simulink model "Control_try_final_2020b"  (R2020b)
settings: Solver=VariableStepAuto  StartTime=0.0  StopTime=inf  RelTol=1e-3
undefined symbols (not defined in the file or in its folder): DiscIntNeverNeededParam
libraries: mobileRoboticsLib x25
(part 2 of 7)

== system Control_try_final_2020b/Team_1_behaviour/T1R2 (attacker 1) ==
  R_1_loc : Inport
  R_2_loc : Inport  Port=2
  R_4_loc : Inport  Port=3
  R_3_loc : Inport  Port=4
  Ball Loc : Inport  Port=5
  R_2_sen : Inport  Port=6
  reset : Inport  Port=7
  did_goal : Inport  Port=8
  foul_team_right : Inport  Port=9
  foul_team_left : Inport  Port=10
  throwin_foul_loc : Inport  Port=11
  Chart1 : Stateflow chart  TreatAsAtomicUnit=on
      settings: PortSchema="{\"entries\":[{\"content\":{\"sides\":[{\"content\":{\"connectorIds\":[\"In8\",\"In2\",\"In3\",\"In4\",\"In5\",\"In6\",\"In7\",\"In9\"]},\"type\":\"ConnectorPlacement.EquallySpacedRectSide\",\"uuid\":\"fbe3839a-d39c-4c99-9a0b-e35240c09fc7\"},{\"content\":{\"connectorIds\":[\"Out1\",\"Out2\",\"Out3\"],\"side\":\"RIGHT\"},\"type\":\"ConnectorPlacement.EquallySpacedRectSide\",\"uuid\":\"d50292e7-ec87-4cb2-bfda-821c8e119e63\"},{\"content\":{\"connectorIds\":[\"In1\"],\"side\":\"TOP\"},\"type\":\"ConnectorPlacement.EquallySpacedRectSide\",\"uuid\":\"096c229a-97d6-46f3-b3a2-f22035fee078\"}]},\"type\":\"ConnectorPlacement.EquallySpacedConnector\",\"uuid\":\"90e2ed61-57b9-4a5d-b9f9-31cf1ac9de3f\"}],\"packageUris\":[\"http://schema.mathworks.com/mf0/Connector/R2020b\"],\"version\":\"1.0\"}"
  Demux : Demux  Outputs=3
  Demux1 : Demux  Outputs=2
  IC1 : InitialCondition  Value=[0;0;0]
  Team 1 Behaviour1 : Subsystem
      settings: PortSchema="{\"entries\":[{\"content\":{\"sides\":[{\"content\":{\"connectorIds\":[]},\"type\":\"ConnectorPlacement.EquallySpacedRectSide\",\"uuid\":\"be901545-21b9-45e5-bac5-a8cb9027aef5\"},{\"content\":{\"connectorIds\":[\"In1\",\"In2\",\"In3\",\"Out1\",\"Out2\",\"In4\",\"In5\",\"In6\",\"In7\",\"In8\"],\"side\":\"RIGHT\"},\"type\":\"ConnectorPlacement.EquallySpacedRectSide\",\"uuid\":\"b7c1eb84-2f14-4c7f-a74c-d56efbe0743e\"},{\"content\":{\"connectorIds\":[],\"side\":\"TOP\"},\"type\":\"ConnectorPlacement.EquallySpacedRectSide\",\"uuid\":\"aca41723-ed3f-4bd2-8fc1-457d075e3460\"}]},\"type\":\"ConnectorPlacement.EquallySpacedConnector\",\"uuid\":\"e10e22f1-c8f0-4dfc-85d2-4ba01528372d\"}],\"packageUris\":[\"http://schema.mathworks.com/mf0/Connector/R2020b\"],\"version\":\"1.0\"}"
  VxVyW : Outport
  XYZK : Outport  Port=2
  wires:
  R_2_sen/1 -> Team 1 Behaviour1/5(Robot 7 sens)
  R_4_loc/1 -> Team 1 Behaviour1/7(Robot 6 T1 Loc3)
  R_1_loc/1 -> Team 1 Behaviour1/8(Robot 5 T1 Loc4)
  R_3_loc/1 -> Team 1 Behaviour1/6(Robot 8 T1 Loc2)
  Demux1/2 -> Chart1/7(foul_loc_y)
  R_2_loc/1 -> Team 1 Behaviour1/4(Robot 1 T1 Loc), Chart1/1(R_2_loc)
  Demux1/1 -> Chart1/6(foul_loc_x)
  Demux/1 -> Chart1/2(bx)
  throwin_foul_loc/1 -> Demux1/1
  Ball Loc/1 -> Demux/1
  foul_team_left/1 -> Chart1/5(foul_team_left)
  did_goal/1 -> Chart1/9(did_goal)
  foul_team_right/1 -> Chart1/4(foul_team_right)
  Demux/2 -> Chart1/3(by)
  Chart1/3(velocity_UA) -> Team 1 Behaviour1/1(velocity_UA)
  Team 1 Behaviour1/1(XYZK) -> XYZK/1
  reset/1 -> Chart1/8(reset)
  Chart1/1(dest) -> IC1/1
  IC1/1 -> Team 1 Behaviour1/3(Ball Loc)
  Team 1 Behaviour1/2(VxVyW) -> VxVyW/1
  Chart1/2(kick_UA) -> Team 1 Behaviour1/2(kick_UA)

== system Control_try_final_2020b/Team_1_behaviour/T1R3 (Defender 2) ==
  R_1_loc : Inport
  R_2_loc : Inport  Port=2
  R_4_loc : Inport  Port=3
  R_3_loc : Inport  Port=4
  Ball Loc : Inport  Port=5
  reset : Inport  Port=6
  R_4_sen : Inport  Port=7
  did_goal : Inport  Port=8
  foul_team_right : Inport  Port=9
  foul_team_left : Inport  Port=10
  throwin_foul_loc : Inport  Port=11
  Chart : Stateflow chart  TreatAsAtomicUnit=on
      settings: PortSchema="{\"entries\":[{\"content\":{\"sides\":[{\"content\":{\"connectorIds\":[\"In9\",\"In2\",\"In3\",\"In4\",\"In5\",\"In6\",\"In7\",\"In8\"]},\"type\":\"ConnectorPlacement.EquallySpacedRectSide\",\"uuid\":\"fbe3839a-d39c-4c99-9a0b-e35240c09fc7\"},{\"content\":{\"connectorIds\":[\"Out1\",\"Out2\",\"Out3\"],\"side\":\"RIGHT\"},\"type\":\"ConnectorPlacement.EquallySpacedRectSide\",\"uuid\":\"d50292e7-ec87-4cb2-bfda-821c8e119e63\"},{\"content\":{\"connectorIds\":[\"In1\"],\"side\":\"TOP\"},\"type\":\"ConnectorPlacement.EquallySpacedRectSide\",\"uuid\":\"096c229a-97d6-46f3-b3a2-f22035fee078\"}]},\"type\":\"ConnectorPlacement.EquallySpacedConnector\",\"uuid\":\"90e2ed61-57b9-4a5d-b9f9-31cf1ac9de3f\"}],\"packageUris\":[\"http://schema.mathworks.com/mf0/Connector/R2020b\"],\"version\":\"1.0\"}"
  Demux : Demux  Outputs=3
  Demux1 : Demux  Outputs=2
  IC : InitialCondition  Value=[0;0;0]
  Team 1 Behaviour1 : Subsystem
      settings: PortSchema="{\"entries\":[{\"content\":{\"sides\":[{\"content\":{\"connectorIds\":[]},\"type\":\"ConnectorPlacement.EquallySpacedRectSide\",\"uuid\":\"be901545-21b9-45e5-bac5-a8cb9027aef5\"},{\"content\":{\"connectorIds\":[\"In1\",\"In2\",\"In3\",\"Out1\",\"Out2\",\"In4\",\"In5\",\"In6\",\"In7\",\"In8\"],\"side\":\"RIGHT\"},\"type\":\"ConnectorPlacement.EquallySpacedRectSide\",\"uuid\":\"b7c1eb84-2f14-4c7f-a74c-d56efbe0743e\"},{\"content\":{\"connectorIds\":[],\"side\":\"TOP\"},\"type\":\"ConnectorPlacement.EquallySpacedRectSide\",\"uuid\":\"aca41723-ed3f-4bd2-8fc1-457d075e3460\"}]},\"type\":\"ConnectorPlacement.EquallySpacedConnector\",\"uuid\":\"e10e22f1-c8f0-4dfc-85d2-4ba01528372d\"}],\"packageUris\":[\"http://schema.mathworks.com/mf0/Connector/R2020b\"],\"version\":\"1.0\"}"
  XYZK : Outport
  Out2 : Outport  Port=2
  wires:
  R_4_sen/1 -> Team 1 Behaviour1/5(Robot 7 sens)
  R_2_loc/1 -> Team 1 Behaviour1/7(Robot 6 T1 Loc3)
  R_3_loc/1 -> Team 1 Behaviour1/6(Robot 8 T1 Loc2)
  R_1_loc/1 -> Team 1 Behaviour1/8(Robot 5 T1 Loc4)
  foul_team_right/1 -> Chart/4(foul_team_right)
  throwin_foul_loc/1 -> Demux1/1
  Demux1/2 -> Chart/8(foul_loc_y)
  Demux1/1 -> Chart/7(foul_loc_x)
  did_goal/1 -> Chart/6(did_goal)
  foul_team_left/1 -> Chart/5(foul_team_left)
  Demux/2 -> Chart/3(by)
  Chart/3(velocity_UA) -> Team 1 Behaviour1/1(velocity_UA)
  Chart/1(dest) -> IC/1
  Chart/2(kick_UA) -> Team 1 Behaviour1/2(kick_UA)
  Team 1 Behaviour1/2(VxVyW) -> XYZK/1
  Demux/1 -> Chart/2(bx)
  IC/1 -> Team 1 Behaviour1/3(Ball Loc)
  Team 1 Behaviour1/1(XYZK) -> Out2/1
  reset/1 -> Chart/9(reset)
  R_4_loc/1 -> Team 1 Behaviour1/4(Robot 1 T1 Loc), Chart/1(R_2_loc)
  Ball Loc/1 -> Demux/1

== system Control_try_final_2020b/Team_1_behaviour/T1R3 (defender 1) ==
  R_1_loc : Inport
  R_2_loc : Inport  Port=2
  R_4_loc : Inport  Port=3
  R_3_loc : Inport  Port=4
  Ball Loc : Inport  Port=5
  reset : Inport  Port=6
  R_3_sen : Inport  Port=7
  did_goal : Inport  Port=8
  foul_team_right : Inport  Port=9
  foul_team_left : Inport  Port=10
  throwin_foul_loc : Inport  Port=11
  Chart : Stateflow chart  TreatAsAtomicUnit=on
      settings: PortSchema="{\"entries\":[{\"content\":{\"sides\":[{\"content\":{\"connectorIds\":[\"In8\",\"In2\",\"In3\",\"In4\",\"In5\",\"In6\",\"In7\",\"In9\"]},\"type\":\"ConnectorPlacement.EquallySpacedRectSide\",\"uuid\":\"fbe3839a-d39c-4c99-9a0b-e35240c09fc7\"},{\"content\":{\"connectorIds\":[\"Out1\",\"Out2\",\"Out3\"],\"side\":\"RIGHT\"},\"type\":\"ConnectorPlacement.EquallySpacedRectSide\",\"uuid\":\"d50292e7-ec87-4cb2-bfda-821c8e119e63\"},{\"content\":{\"connectorIds\":[\"In1\"],\"side\":\"TOP\"},\"type\":\"ConnectorPlacement.EquallySpacedRectSide\",\"uuid\":\"096c229a-97d6-46f3-b3a2-f22035fee078\"},{\"content\":{\"connectorIds\":[],\"side\":\"BOTTOM\"},\"type\":\"ConnectorPlacement.EquallySpacedRectSide\",\"uuid\":\"82b7a600-d24c-4262-afa5-d1d8e08c64b1\"}]},\"type\":\"ConnectorPlacement.EquallySpacedConnector\",\"uuid\":\"90e2ed61-57b9-4a5d-b9f9-31cf1ac9de3f\"}],\"packageUris\":[\"http://schema.mathworks.com/mf0/Connector/R2020b\"],\"version\":\"1.0\"}"
  Demux : Demux  Outputs=3
  Demux1 : Demux  Outputs=2
  IC : InitialCondition  Value=[0;0;0]
  Team 1 Behaviour : Subsystem  Commented=on
      settings: PortSchema="{\"entries\":[{\"content\":{\"sides\":[{\"content\":{\"connectorIds\":[]},\"type\":\"ConnectorPlacement.EquallySpacedRectSide\",\"uuid\":\"be901545-21b9-45e5-bac5-a8cb9027aef5\"},{\"content\":{\"connectorIds\":[\"In1\",\"Out1\",\"Out2\",\"In2\"],\"side\":\"RIGHT\"},\"type\":\"ConnectorPlacement.EquallySpacedRectSide\",\"uuid\":\"b7c1eb84-2f14-4c7f-a74c-d56efbe0743e\"},{\"content\":{\"connectorIds\":[],\"side\":\"TOP\"},\"type\":\"ConnectorPlacement.EquallySpacedRectSide\",\"uuid\":\"aca41723-ed3f-4bd2-8fc1-457d075e3460\"}]},\"type\":\"ConnectorPlacement.EquallySpacedConnector\",\"uuid\":\"e10e22f1-c8f0-4dfc-85d2-4ba01528372d\"}],\"packageUris\":[\"http://schema.mathworks.com/mf0/Connector/R2020b\"],\"version\":\"1.0\"}"
  Team 1 Behaviour1 : Subsystem
      settings: PortSchema="{\"entries\":[{\"content\":{\"sides\":[{\"content\":{\"connectorIds\":[]},\"type\":\"ConnectorPlacement.EquallySpacedRectSide\",\"uuid\":\"be901545-21b9-45e5-bac5-a8cb9027aef5\"},{\"content\":{\"connectorIds\":[\"In1\",\"In2\",\"In3\",\"Out1\",\"Out2\",\"In4\",\"In5\",\"In6\",\"In7\",\"In8\"],\"side\":\"RIGHT\"},\"type\":\"ConnectorPlacement.EquallySpacedRectSide\",\"uuid\":\"b7c1eb84-2f14-4c7f-a74c-d56efbe0743e\"},{\"content\":{\"connectorIds\":[],\"side\":\"TOP\"},\"type\":\"ConnectorPlacement.EquallySpacedRectSide\",\"uuid\":\"aca41723-ed3f-4bd2-8fc1-457d075e3460\"}]},\"type\":\"ConnectorPlacement.EquallySpacedConnector\",\"uuid\":\"e10e22f1-c8f0-4dfc-85d2-4ba01528372d\"}],\"packageUris\":[\"http://schema.mathworks.com/mf0/Connector/R2020b\"],\"version\":\"1.0\"}"
  VxVyW : Outport
  XYZK : Outport  Port=2
  wires:
  reset/1 -> Chart/8(reset)
  Ball Loc/1 -> Demux/1
  Demux/1 -> Chart/2(bx)
  Team 1 Behaviour1/2(VxVyW) -> VxVyW/1
  Team 1 Behaviour1/1(XYZK) -> XYZK/1
  R_3_loc/1 -> Team 1 Behaviour1/4(Robot 1 T1 Loc), Chart/1(R_2_loc)
  Demux/2 -> Chart/3(by)
  Chart/1(dest) -> IC/1
  IC/1 -> Team 1 Behaviour1/3(Ball Loc)
  Chart/2(kick_UA) -> Team 1 Behaviour1/2(kick_UA)
  Chart/3(velocity_UA) -> Team 1 Behaviour1/1(velocity_UA)
  did_goal/1 -> Chart/9(did_goal)
  foul_team_right/1 -> Chart/7(foul_team_right)
  foul_team_left/1 -> Chart/4(foul_team_left)
  throwin_foul_loc/1 -> Demux1/1
  Demux1/1 -> Chart/5(foul_loc_x)
  Demux1/2 -> Chart/6(foul_loc_y)
  R_1_loc/1 -> Team 1 Behaviour1/8(Robot 5 T1 Loc4)
  R_3_sen/1 -> Team 1 Behaviour1/5(Robot 7 sens)
  R_2_loc/1 -> Team 1 Behaviour1/7(Robot 6 T1 Loc3)
  R_4_loc/1 -> Team 1 Behaviour1/6(Robot 8 T1 Loc2)

== system Control_try_final_2020b/Team_2_Behaviour/T2_R1(Goal_Keeper) ==
  R_1_loc : Inport
  R_2_loc : Inport  Port=2
  R_4_loc : Inport  Port=3
  R_3_loc : Inport  Port=4
  Ball Loc : Inport  Port=5
  R_1_sen : Inport  Port=6
  Constant : Constant  Value=0
  Constant1 : Constant  Value=0
  Demux : Demux  Outputs=3
  Demux1 : Demux  Outputs=3
  Display : Display
  Distance : Subsystem
      settings: PortSchema="{\"entries\":[{\"content\":{\"sides\":[{\"content\":{\"connectorIds\":[]},\"type\":\"ConnectorPlacement.EquallySpacedRectSide\",\"uuid\":\"931fdb8b-3711-4e7f-9cbc-53e0dea53fca\"},{\"content\":{\"connectorIds\":[\"Out1\"],\"side\":\"RIGHT\"},\"type\":\"ConnectorPlacement.EquallySpacedRectSide\",\"uuid\":\"ee0c7800-c700-48d1-aa4f-dd4a30624bbc\"},{\"content\":{\"connectorIds\":[\"In1\",\"In2\"],\"side\":\"TOP\"},\"type\":\"ConnectorPlacement.EquallySpacedRectSide\",\"uuid\":\"9579cc4b-8b33-4755-9564-e19cfe104d2b\"},{\"content\":{\"connectorIds\":[\"In3\",\"In4\"],\"side\":\"BOTTOM\"},\"type\":\"ConnectorPlacement.EquallySpacedRectSide\",\"uuid\":\"3469c1a3-363b-4534-8624-9a42e1898f6f\"}]},\"type\":\"ConnectorPlacement.EquallySpacedConnector\",\"uuid\":\"efd995f2-e999-4310-9f3f-88c38333e880\"}],\"packageUris\":[\"http://schema.mathworks.com/mf0/Connector/R2020b\"],\"version\":\"1.0\"}"
  Vector Concatenate : Concatenate  NumInputs=3
  angle_finder : Subsystem
  control : Stateflow chart  TreatAsAtomicUnit=on
      settings: PortSchema="{\"entries\":[{\"content\":{\"sides\":[{\"content\":{\"connectorIds\":[\"In1\",\"In4\",\"In3\",\"In2\",\"In5\"]},\"type\":\"ConnectorPlacement.EquallySpacedRectSide\",\"uuid\":\"fa0fd246-e6b9-4dd4-94af-e6e1e45d6f7d\"},{\"content\":{\"connectorIds\":[\"Out1\",\"Out2\"],\"side\":\"RIGHT\"},\"type\":\"ConnectorPlacement.EquallySpacedRectSide\",\"uuid\":\"3f196244-96d1-41e4-aa84-a415e0f99109\"},{\"content\":{\"connectorIds\":[],\"side\":\"TOP\"},\"type\":\"ConnectorPlacement.EquallySpacedRectSide\",\"uuid\":\"731ebc3a-62ab-4275-8d10-19257bb8fb52\"}]},\"type\":\"ConnectorPlacement.EquallySpacedConnector\",\"uuid\":\"dccf28de-3df1-4952-8544-1d4b47a347e5\"}],\"packageUris\":[\"http://schema.mathworks.com/mf0/Connector/R2020b\"],\"version\":\"1.0\"}"
  min_Distance_Finder : Subsystem
      settings: PortSchema="{\"entries\":[{\"content\":{\"sides\":[{\"content\":{\"connectorIds\":[\"In1\",\"In2\"]},\"type\":\"ConnectorPlacement.EquallySpacedRectSide\",\"uuid\":\"45cf91c7-7d38-4a19-bf35-d1d31095287a\"},{\"content\":{\"connectorIds\":[\"Out1\"],\"side\":\"RIGHT\"},\"type\":\"ConnectorPlacement.EquallySpacedRectSide\",\"uuid\":\"645394ba-2e5d-4060-b61c-cc9330ee0038\"},{\"content\":{\"connectorIds\":[\"In3\",\"In4\",\"In5\"],\"side\":\"TOP\"},\"type\":\"ConnectorPlacement.EquallySpacedRectSide\",\"uuid\":\"4fc56b73-04ec-476f-b487-f0e593f708ad\"},{\"content\":{\"connectorIds\":[],\"side\":\"BOTTOM\"},\"type\":\"ConnectorPlacement.EquallySpacedRectSide\",\"uuid\":\"cd306436-fd63-4e79-88e6-7a63c0840ed7\"}]},\"type\":\"ConnectorPlacement.EquallySpacedConnector\",\"uuid\":\"5cf2ee04-00eb-490b-958c-5fb90b43d325\"}],\"packageUris\":[\"http://schema.mathworks.com/mf0/Connector/R2020b\"],\"version\":\"1.0\"}"
  R1_vel_Y : Outport
  kick : Outport  Port=2  PortDimensions=4
  wires:
  Ball Loc/1 -> Demux/1
  Demux/2 -> control/5(Ball_loc_Y), Distance/4(In4)
  R_1_loc/1 -> Demux1/1, angle_finder/2(R_1_loc), min_Distance_Finder/2(R_1_loc)
  Demux1/2 -> control/4(R1_loc_Y), Distance/2(In2)
  Demux1/1 -> control/1(R1_loc_X), Distance/1(In1)
  R_2_loc/1 -> min_Distance_Finder/3(R_2_loc)
  R_3_loc/1 -> min_Distance_Finder/4(R_3_loc)
  R_4_loc/1 -> min_Distance_Finder/5(R_4_loc)
  R_1_sen/1 -> min_Distance_Finder/1(R_1_sen)
  Demux/1 -> control/2(Ball_loc_X), Distance/3(In3)
  control/2(R1_vel_Y) -> Vector Concatenate/2
  Distance/1(GB_dist) -> control/3(GB_dist)
  Vector Concatenate/1 -> R1_vel_Y/1
  Constant/1 -> Vector Concatenate/1
  Constant1/1 -> Vector Concatenate/3
  min_Distance_Finder/1(kick_direction) -> angle_finder/1(kick_direction)
  control/1(kick) -> angle_finder/3(kick)
  angle_finder/1(Out1) -> Display/1, kick/1

== system Control_try_final_2020b/Team_2_Behaviour/T2_R2(defender) ==
  R_1_loc : Inport
  R_2_loc : Inport  Port=2
  R_4_loc : Inport  Port=3
  R_3_loc : Inport  Port=4
  Ball Loc : Inport  Port=5
  reset : Inport  Port=6
  R_2_sen : Inport  Port=7
  did_goal : Inport  Port=8
  foul_team_right : Inport  Port=9
  foul_team_left : Inport  Port=10
  throwin_foul_loc : Inport  Port=11
  Chart : Stateflow chart  TreatAsAtomicUnit=on
      settings: PortSchema="{\"entries\":[{\"content\":{\"sides\":[{\"content\":{\"connectorIds\":[\"In9\",\"In2\",\"In3\",\"In4\",\"In5\",\"In6\",\"In7\",\"In8\"]},\"type\":\"ConnectorPlacement.EquallySpacedRectSide\",\"uuid\":\"fbe3839a-d39c-4c99-9a0b-e35240c09fc7\"},{\"content\":{\"connectorIds\":[\"Out1\",\"Out2\",\"Out3\"],\"side\":\"RIGHT\"},\"type\":\"ConnectorPlacement.EquallySpacedRectSide\",\"uuid\":\"d50292e7-ec87-4cb2-bfda-821c8e119e63\"},{\"content\":{\"connectorIds\":[\"In1\"],\"side\":\"TOP\"},\"type\":\"ConnectorPlacement.EquallySpacedRectSide\",\"uuid\":\"096c229a-97d6-46f3-b3a2-f22035fee078\"}]},\"type\":\"ConnectorPlacement.EquallySpacedConnector\",\"uuid\":\"90e2ed61-57b9-4a5d-b9f9-31cf1ac9de3f\"}],\"packageUris\":[\"http://schema.mathworks.com/mf0/Connector/R2020b\"],\"version\":\"1.0\"}"
  Demux : Demux  Outputs=3
  Demux1 : Demux  Outputs=2
  IC : InitialCondition  Value=[0;0;0]
  Team 1 Behaviour1 : Subsystem
      settings: PortSchema="{\"entries\":[{\"content\":{\"sides\":[{\"content\":{\"connectorIds\":[]},\"type\":\"ConnectorPlacement.EquallySpacedRectSide\",\"uuid\":\"be901545-21b9-45e5-bac5-a8cb9027aef5\"},{\"content\":{\"connectorIds\":[\"In1\",\"In2\",\"In3\",\"Out1\",\"Out2\",\"In4\",\"In5\",\"In6\",\"In7\",\"In8\"],\"side\":\"RIGHT\"},\"type\":\"ConnectorPlacement.EquallySpacedRectSide\",\"uuid\":\"b7c1eb84-2f14-4c7f-a74c-d56efbe0743e\"},{\"content\":{\"connectorIds\":[],\"side\":\"TOP\"},\"type\":\"ConnectorPlacement.EquallySpacedRectSide\",\"uuid\":\"aca41723-ed3f-4bd2-8fc1-457d075e3460\"}]},\"type\":\"ConnectorPlacement.EquallySpacedConnector\",\"uuid\":\"e10e22f1-c8f0-4dfc-85d2-4ba01528372d\"}],\"packageUris\":[\"http://schema.mathworks.com/mf0/Connector/R2020b\"],\"version\":\"1.0\"}"
  VxVyW : Outport
  XYZK : Outport  Port=2
  wires:
  throwin_foul_loc/1 -> Demux1/1
  Demux1/1 -> Chart/4(foul_loc_x)
  R_3_loc/1 -> Team 1 Behaviour1/6(Robot 8 T1 Loc2)
  R_4_loc/1 -> Team 1 Behaviour1/7(Robot 6 T1 Loc3)
  R_2_sen/1 -> Team 1 Behaviour1/5(Robot 7 sens)
  R_1_loc/1 -> Team 1 Behaviour1/8(Robot 5 T1 Loc4)
  foul_team_right/1 -> Chart/7(foul_team_right)
  Demux1/2 -> Chart/5(foul_loc_y)
  foul_team_left/1 -> Chart/6(foul_team_left)
  Chart/3(velocity_UA) -> Team 1 Behaviour1/1(velocity_UA)
  did_goal/1 -> Chart/8(did_goal)
  reset/1 -> Chart/9(reset)
  Chart/2(kick_UA) -> Team 1 Behaviour1/2(kick_unactivate)
  IC/1 -> Team 1 Behaviour1/3(Ball Loc)
  Chart/1(dest) -> IC/1
  Demux/2 -> Chart/3(by)
  Team 1 Behaviour1/1(XYZK) -> XYZK/1
  Team 1 Behaviour1/2(VxVyW) -> VxVyW/1
  Demux/1 -> Chart/2(bx)
  Ball Loc/1 -> Demux/1
  R_2_loc/1 -> Team 1 Behaviour1/4(Robot 1 T1 Loc), Chart/1(R_2_loc)

== system Control_try_final_2020b/Team_2_Behaviour/T2_R3(Attacker 1) ==
  R_1_loc : Inport
  R_2_loc : Inport  Port=2
  R_4_loc : Inport  Port=3
  R_3_loc : Inport  Port=4
  Ball Loc : Inport  Port=5
  reset : Inport  Port=6
  R_3_sen : Inport  Port=7
  did_goal : Inport  Port=8
  foul_team_right : Inport  Port=9
  foul_team_left : Inport  Port=10
  throwin_foul_loc : Inport  Port=11
  Chart : Stateflow chart  TreatAsAtomicUnit=on
      settings: PortSchema="{\"entries\":[{\"content\":{\"sides\":[{\"content\":{\"connectorIds\":[\"In9\",\"In2\",\"In3\",\"In4\",\"In5\",\"In6\",\"In7\",\"In8\"]},\"type\":\"ConnectorPlacement.EquallySpacedRectSide\",\"uuid\":\"fbe3839a-d39c-4c99-9a0b-e35240c09fc7\"},{\"content\":{\"connectorIds\":[\"Out1\",\"Out2\",\"Out3\"],\"side\":\"RIGHT\"},\"type\":\"ConnectorPlacement.EquallySpacedRectSide\",\"uuid\":\"d50292e7-ec87-4cb2-bfda-821c8e119e63\"},{\"content\":{\"connectorIds\":[\"In1\"],\"side\":\"TOP\"},\"type\":\"ConnectorPlacement.EquallySpacedRectSide\",\"uuid\":\"096c229a-97d6-46f3-b3a2-f22035fee078\"}]},\"type\":\"ConnectorPlacement.EquallySpacedConnector\",\"uuid\":\"90e2ed61-57b9-4a5d-b9f9-31cf1ac9de3f\"}],\"packageUris\":[\"http://schema.mathworks.com/mf0/Connector/R2020b\"],\"version\":\"1.0\"}"
  Demux : Demux  Outputs=3
  Demux1 : Demux  Outputs=2
  IC : InitialCondition  Value=[0;0;0]
  Team 1 Behaviour1 : Subsystem
      settings: PortSchema="{\"entries\":[{\"content\":{\"sides\":[{\"content\":{\"connectorIds\":[]},\"type\":\"ConnectorPlacement.EquallySpacedRectSide\",\"uuid\":\"be901545-21b9-45e5-bac5-a8cb9027aef5\"},{\"content\":{\"connectorIds\":[\"In1\",\"In2\",\"In3\",\"Out1\",\"Out2\",\"In4\",\"In5\",\"In6\",\"In7\",\"In8\"],\"side\":\"RIGHT\"},\"type\":\"ConnectorPlacement.EquallySpacedRectSide\",\"uuid\":\"b7c1eb84-2f14-4c7f-a74c-d56efbe0743e\"},{\"content\":{\"connectorIds\":[],\"side\":\"TOP\"},\"type\":\"ConnectorPlacement.EquallySpacedRectSide\",\"uuid\":\"aca41723-ed3f-4bd2-8fc1-457d075e3460\"}]},\"type\":\"ConnectorPlacement.EquallySpacedConnector\",\"uuid\":\"e10e22f1-c8f0-4dfc-85d2-4ba01528372d\"}],\"packageUris\":[\"http://schema.mathworks.com/mf0/Connector/R2020b\"],\"version\":\"1.0\"}"
  VxVyW : Outport
  XYZK : Outport  Port=2
  wires:
  R_3_sen/1 -> Team 1 Behaviour1/5(Robot 7 sens)
  R_4_loc/1 -> Team 1 Behaviour1/6(Robot 8 T1 Loc2)
  R_2_loc/1 -> Team 1 Behaviour1/7(Robot 6 T1 Loc3)
  R_1_loc/1 -> Team 1 Behaviour1/8(Robot 5 T1 Loc4)
  foul_team_right/1 -> Chart/7(foul_team_right)
  Demux1/2 -> Chart/5(foul_loc_y)
  did_goal/1 -> Chart/8(did_goal)
  foul_team_left/1 -> Chart/6(foul_team_left)
  Demux1/1 -> Chart/4(foul_loc_x)
  throwin_foul_loc/1 -> Demux1/1
  Chart/3(velocity_UA) -> Team 1 Behaviour1/1(velocity_UA)
  Chart/2(kick_UA) -> Team 1 Behaviour1/2(kick_UA)
  Demux/1 -> Chart/2(bx)
  Ball Loc/1 -> Demux/1
  Demux/2 -> Chart/3(by)
  Team 1 Behaviour1/2(VxVyW) -> VxVyW/1
  IC/1 -> Team 1 Behaviour1/3(Ball Loc)
  Chart/1(dest) -> IC/1
  Team 1 Behaviour1/1(XYZK) -> XYZK/1
  reset/1 -> Chart/9(reset)
  R_3_loc/1 -> Team 1 Behaviour1/4(Robot 1 T1 Loc), Chart/1(R_2_loc)

== system Control_try_final_2020b/Team_2_Behaviour/T3_R4(Attacker 2) ==
  R_1_loc : Inport
  R_2_loc : Inport  Port=2
  R_4_loc : Inport  Port=3
  R_3_loc : Inport  Port=4
  Ball Loc : Inport  Port=5
  reset : Inport  Port=6
  R_4_sen : Inport  Port=7
  did_goal : Inport  Port=8
  foul_team_right : Inport  Port=9
  foul_team_left : Inport  Port=10
  CFL : Inport  Port=11
  CFR : Inport  Port=12
  C_foul_loc : Inport  Port=13
  throwin_foul_loc : Inport  Port=14
  Chart : Stateflow chart  TreatAsAtomicUnit=on
      settings: PortSchema="{\"entries\":[{\"content\":{\"sides\":[{\"content\":{\"connectorIds\":[\"In13\",\"In2\",\"In3\",\"In4\",\"In5\",\"In6\",\"In7\",\"In8\",\"In9\",\"In10\",\"In11\",\"In12\"]},\"type\":\"ConnectorPlacement.EquallySpacedRectSide\",\"uuid\":\"fbe3839a-d39c-4c99-9a0b-e35240c09fc7\"},{\"content\":{\"connectorIds\":[\"Out1\",\"Out2\",\"Out3\"],\"side\":\"RIGHT\"},\"type\":\"ConnectorPlacement.EquallySpacedRectSide\",\"uuid\":\"d50292e7-ec87-4cb2-bfda-821c8e119e63\"},{\"content\":{\"connectorIds\":[\"In1\"],\"side\":\"TOP\"},\"type\":\"ConnectorPlacement.EquallySpacedRectSide\",\"uuid\":\"096c229a-97d6-46f3-b3a2-f22035fee078\"}]},\"type\":\"ConnectorPlacement.EquallySpacedConnector\",\"uuid\":\"90e2ed61-57b9-4a5d-b9f9-31cf1ac9de3f\"}],\"packageUris\":[\"http://schema.mathworks.com/mf0/Connector/R2020b\"],\"version\":\"1.0\"}"
  Demux : Demux  Outputs=3
  Demux1 : Demux  Outputs=2
  Demux2 : Demux  Outputs=2
  IC : InitialCondition  Value=[0;0;0]
  Team 1 Behaviour1 : Subsystem
      settings: PortSchema="{\"entries\":[{\"content\":{\"sides\":[{\"content\":{\"connectorIds\":[]},\"type\":\"ConnectorPlacement.EquallySpacedRectSide\",\"uuid\":\"be901545-21b9-45e5-bac5-a8cb9027aef5\"},{\"content\":{\"connectorIds\":[\"In1\",\"In2\",\"In3\",\"Out1\",\"Out2\",\"In4\",\"In5\",\"In6\",\"In7\",\"In8\"],\"side\":\"RIGHT\"},\"type\":\"ConnectorPlacement.EquallySpacedRectSide\",\"uuid\":\"b7c1eb84-2f14-4c7f-a74c-d56efbe0743e\"},{\"content\":{\"connectorIds\":[],\"side\":\"TOP\"},\"type\":\"ConnectorPlacement.EquallySpacedRectSide\",\"uuid\":\"aca41723-ed3f-4bd2-8fc1-457d075e3460\"}]},\"type\":\"ConnectorPlacement.EquallySpacedConnector\",\"uuid\":\"e10e22f1-c8f0-4dfc-85d2-4ba01528372d\"}],\"packageUris\":[\"http://schema.mathworks.com/mf0/Connector/R2020b\"],\"version\":\"1.0\"}"
  XYZK : Outport
  Out2 : Outport  Port=2
  wires:
  R_4_sen/1 -> Team 1 Behaviour1/5(Robot 7 sens)
  R_3_loc/1 -> Team 1 Behaviour1/6(Robot 8 T1 Loc2)
  R_2_loc/1 -> Team 1 Behaviour1/7(Robot 6 T1 Loc3)
  R_1_loc/1 -> Team 1 Behaviour1/8(Robot 5 T1 Loc4)
  Demux2/1 -> Chart/11(C_foul_loc_x)
  R_4_loc/1 -> Team 1 Behaviour1/4(Robot 1 T1 Loc), Chart/1(R_2_loc)
  Demux2/2 -> Chart/12(C_foul_loc_y)
  Team 1 Behaviour1/2(VxVyW) -> XYZK/1
  C_foul_loc/1 -> Demux2/1
  reset/1 -> Chart/13(reset)
  CFR/1 -> Chart/10(CFR)
  did_goal/1 -> Chart/8(did_goal)
  CFL/1 -> Chart/9(CFL)
  Ball Loc/1 -> Demux/1
  Demux1/2 -> Chart/5(foul_loc_y)
  foul_team_right/1 -> Chart/7(foul_team_right)
  Demux1/1 -> Chart/4(foul_loc_x)
  throwin_foul_loc/1 -> Demux1/1
  foul_team_left/1 -> Chart/6(foul_team_left)
  Team 1 Behaviour1/1(XYZK) -> Out2/1
  Chart/3(velocity_UA) -> Team 1 Behaviour1/1(velocity_UA)
  IC/1 -> Team 1 Behaviour1/3(Ball Loc)
  Chart/2(kick_UA) -> Team 1 Behaviour1/2(kick_UA)
  Demux/2 -> Chart/3(by)
  Demux/1 -> Chart/2(bx)
  Chart/1(dest) -> IC/1

== system Control_try_final_2020b/Team_1_behaviour/T1R1(Goal_Keeper)/Ball_in_D ==
  Ball Loc : Inport
  Robot 1 T1 Loc : Inport  Port=2
  In1 : Inport  Port=3
  Angle Finder : Subsystem
  Chart : Stateflow chart  TreatAsAtomicUnit=on
      settings: PortSchema="{\"entries\":[{\"content\":{\"sides\":[{\"content\":{\"connectorIds\":[\"In5\",\"In1\",\"In2\",\"In3\",\"In4\",\"In6\"]},\"type\":\"ConnectorPlacement.EquallySpacedRectSide\",\"uuid\":\"cd25ea97-6441-4246-83f2-eec847899c89\"},{\"content\":{\"connectorIds\":[\"Out1\"],\"side\":\"RIGHT\"},\"type\":\"ConnectorPlacement.EquallySpacedRectSide\",\"uuid\":\"ef7d77a7-1549-4474-8b84-35bb8af5d0e7\"},{\"content\":{\"connectorIds\":[],\"side\":\"TOP\"},\"type\":\"ConnectorPlacement.EquallySpacedRectSide\",\"uuid\":\"0f0ce596-3061-42ac-890a-62bc4f21ac3e\"},{\"content\":{\"connectorIds\":[],\"side\":\"BOTTOM\"},\"type\":\"ConnectorPlacement.EquallySpacedRectSide\",\"uuid\":\"682b3de5-e999-4954-b7ff-f16ecbf9ea8f\"}]},\"type\":\"ConnectorPlacement.EquallySpacedConnector\",\"uuid\":\"15dca8e2-6a60-4a0d-80a5-3c295a61c828\"}],\"packageUris\":[\"http://schema.mathworks.com/mf0/Connector/R2020b\"],\"version\":\"1.0\"}"
  Chart3 : Stateflow chart  TreatAsAtomicUnit=on
  Constant2 : Constant  Value=2
  Constant3 : Constant  Value=0
  Demux : Demux  Outputs=3
  Demux1 : Demux  Outputs=3
  Demux3 : Demux  Outputs=3
  Matrix Concatenate : Concatenate  Mode=Multidimensional array  ConcatenateDimension=2
  Mod : Math  Operator=mod  SaturateOnIntegerOverflow=on
  Pi : Constant  Value=pi  OutDataTypeStr=Inherit: Inherit via back propagation
  Product1 : Product
  Proximity_Finder_Ball : Subsystem
  Sum : Sum  Inputs=+-
  Sum1 : Sum  Inputs=-+
  Vector Concatenate : Concatenate
  Vector Concatenate1 : Concatenate  NumInputs=3
  Vector Concatenate2 : Concatenate
  Velocity_Decider : Stateflow chart  TreatAsAtomicUnit=on
  kick_direction : Subsystem
  VxVyW : Outport
  XYZK : Outport  Port=2
  wires:
  Ball Loc/1 -> Demux3/1
  Sum/1 -> Proximity_Finder_Ball/1(In1), Angle Finder/1(In1)
  Robot 1 T1 Loc/1 -> Demux1/1
  Demux1/1 -> Matrix Concatenate/1, Chart/3(Rx)
  Demux1/2 -> Matrix Concatenate/2, Chart/4(Ry)
  Matrix Concatenate/1 -> Sum1/2, Sum/1
  Demux3/2 -> Vector Concatenate2/2, Chart/2(By)
  Demux3/1 -> Vector Concatenate2/1, Chart/1(Bx)
  Demux1/3 -> Mod/1
  Pi/1 -> Product1/1
  Constant2/1 -> Product1/2
  Product1/1 -> Mod/2
  Chart/1(actual_angle) -> Chart3/2(DT)
  Mod/1 -> Chart/6(angle_bot)
  Angle Finder/1(angle) -> Chart/5(angle)
  Proximity_Finder_Ball/1(DBR) -> Velocity_Decider/1(DBR)
  Velocity_Decider/2(velocity) -> Chart3/1(velocity)
  Vector Concatenate/1 -> Sum1/1
  Sum1/1 -> kick_direction/1(In1)
  Velocity_Decider/1(kick) -> kick_direction/2(kick)
  kick_direction/1(Out1) -> XYZK/1
  Chart3/1(v) -> Vector Concatenate1/1
  Chart3/2(w) -> Vector Concatenate1/3
  Constant3/1 -> Vector Concatenate1/2
  Vector Concatenate1/1 -> VxVyW/1
  Vector Concatenate2/1 -> Sum/2
  In1/1 -> Demux/1
  Demux/1 -> Vector Concatenate/1
  Demux/2 -> Vector Concatenate/2

== system Control_try_final_2020b/Team_1_behaviour/T1R1(Goal_Keeper)/ball_out_of_D ==
  kick_direction : Inport
  R_1_loc : Inport  Port=2
  Ball Loc : Inport  Port=3
  Constant : Constant  Value=0
  Constant1 : Constant  Value=0
  Demux : Demux  Outputs=3
  Demux1 : Demux  Outputs=3
  Distance : Subsystem
      settings: PortSchema="{\"entries\":[{\"content\":{\"sides\":[{\"content\":{\"connectorIds\":[]},\"type\":\"ConnectorPlacement.EquallySpacedRectSide\",\"uuid\":\"931fdb8b-3711-4e7f-9cbc-53e0dea53fca\"},{\"content\":{\"connectorIds\":[\"Out1\"],\"side\":\"RIGHT\"},\"type\":\"ConnectorPlacement.EquallySpacedRectSide\",\"uuid\":\"ee0c7800-c700-48d1-aa4f-dd4a30624bbc\"},{\"content\":{\"connectorIds\":[\"In1\",\"In2\"],\"side\":\"TOP\"},\"type\":\"ConnectorPlacement.EquallySpacedRectSide\",\"uuid\":\"9579cc4b-8b33-4755-9564-e19cfe104d2b\"},{\"content\":{\"connectorIds\":[\"In3\",\"In4\"],\"side\":\"BOTTOM\"},\"type\":\"ConnectorPlacement.EquallySpacedRectSide\",\"uuid\":\"3469c1a3-363b-4534-8624-9a42e1898f6f\"}]},\"type\":\"ConnectorPlacement.EquallySpacedConnector\",\"uuid\":\"efd995f2-e999-4310-9f3f-88c38333e880\"}],\"packageUris\":[\"http://schema.mathworks.com/mf0/Connector/R2020b\"],\"version\":\"1.0\"}"
  Subsystem : Subsystem
  Vector Concatenate : Concatenate  NumInputs=3
  control : Stateflow chart  TreatAsAtomicUnit=on
      settings: PortSchema="{\"entries\":[{\"content\":{\"sides\":[{\"content\":{\"connectorIds\":[\"In1\",\"In4\",\"In3\",\"In2\",\"In5\"]},\"type\":\"ConnectorPlacement.EquallySpacedRectSide\",\"uuid\":\"fa0fd246-e6b9-4dd4-94af-e6e1e45d6f7d\"},{\"content\":{\"connectorIds\":[\"Out1\",\"Out2\"],\"side\":\"RIGHT\"},\"type\":\"ConnectorPlacement.EquallySpacedRectSide\",\"uuid\":\"3f196244-96d1-41e4-aa84-a415e0f99109\"},{\"content\":{\"connectorIds\":[],\"side\":\"TOP\"},\"type\":\"ConnectorPlacement.EquallySpacedRectSide\",\"uuid\":\"731ebc3a-62ab-4275-8d10-19257bb8fb52\"}]},\"type\":\"ConnectorPlacement.EquallySpacedConnector\",\"uuid\":\"dccf28de-3df1-4952-8544-1d4b47a347e5\"}],\"packageUris\":[\"http://schema.mathworks.com/mf0/Connector/R2020b\"],\"version\":\"1.0\"}"
  Out2 : Outport
  R1_vel_Y : Outport  Port=2
  wires:
  Distance/1(GB_dist) -> control/3(GB_dist)
  Demux/2 -> control/5(Ball_loc_Y), Distance/4(In4)
  Demux/1 -> control/2(Ball_loc_X), Distance/3(In3)
  control/2(R1_vel_Y) -> Vector Concatenate/2
  Constant1/1 -> Vector Concatenate/3
  Demux1/2 -> control/4(R1_loc_Y), Distance/2(In2)
  control/1(kick) -> Subsystem/3(kick)
  Constant/1 -> Vector Concatenate/1
  Demux1/1 -> control/1(R1_loc_X), Distance/1(In1)
  Ball Loc/1 -> Demux/1
  R_1_loc/1 -> Subsystem/2(R_1_loc), Demux1/1
  kick_direction/1 -> Subsystem/1(kick_direction)
  Vector Concatenate/1 -> R1_vel_Y/1
  Subsystem/1(Out1) -> Out2/1

== system Control_try_final_2020b/Team_1_behaviour/T1R1(Goal_Keeper)/min_Distance_Finder ==
  R_1_sen : Inport
  R_1_loc : Inport  Port=2
  R_2_loc : Inport  Port=3
  R_3_loc : Inport  Port=4
  R_4_loc : Inport  Port=5
  Display{,1..2,4} (4 alike) : Display
  Distance : Subsystem
  Distance1 : Subsystem
  Distance2 : Subsystem
  Kick_prob_calc : Stateflow chart  TreatAsAtomicUnit=on
      settings: PortSchema="{\"entries\":[{\"content\":{\"sides\":[{\"content\":{\"connectorIds\":[\"In4\",\"In5\",\"In6\"]},\"type\":\"ConnectorPlacement.EquallySpacedRectSide\",\"uuid\":\"64545375-395a-4478-8a53-b77c7ccd5016\"},{\"content\":{\"connectorIds\":[\"Out1\"],\"side\":\"RIGHT\"},\"type\":\"ConnectorPlacement.EquallySpacedRectSide\",\"uuid\":\"7cc0c28a-cc26-4f23-9952-6261e736221a\"},{\"content\":{\"connectorIds\":[\"In2\",\"In3\",\"In1\"],\"side\":\"TOP\"},\"type\":\"ConnectorPlacement.EquallySpacedRectSide\",\"uuid\":\"3f39c863-1804-4707-87c1-6f77798d874b\"},{\"content\":{\"connectorIds\":[],\"side\":\"BOTTOM\"},\"type\":\"ConnectorPlacement.EquallySpacedRectSide\",\"uuid\":\"dd00a5df-2ac1-49a5-bc9d-cbc3bc53305b\"}]},\"type\":\"ConnectorPlacement.EquallySpacedConnector\",\"uuid\":\"731ad359-9b43-4c19-839e-d6f1a372c8a6\"}],\"packageUris\":[\"http://schema.mathworks.com/mf0/Connector/R2020b\"],\"version\":\"1.0\"}"
  Multiply : Gain  Gain=2
  Multiply1 : Gain  Gain=2
  Multiply2 : Gain  Gain=2
  R2_O_dist_val : Subsystem
  R3_O_dist_val : Subsystem
  R4_O_dist_val : Subsystem
  Sum : Sum  Inputs=|--
  Sum1 : Sum  Inputs=|--
  Sum2 : Sum  Inputs=|--
  zero_padding : MATLAB Function  TreatAsAtomicUnit=on
  kick_direction : Outport
  wires:
  R_2_loc/1 -> R2_O_dist_val/2(R_2_loc), Distance/2(R_2_loc), Kick_prob_calc/2(R_2_loc)
  R_1_loc/1 -> R4_O_dist_val/1(R_1_loc), R3_O_dist_val/1(R_1_loc), R2_O_dist_val/1(R_1_loc), Distance2/1(R_1_loc), Distance1/1(R_1_loc), Distance/1(R_1_loc)
  R_3_loc/1 -> R3_O_dist_val/2(R_2_loc), Distance1/2(R_3_loc), Kick_prob_calc/3(R_3_loc)
  R_4_loc/1 -> R4_O_dist_val/2(R_2_loc), Distance2/2(R_4_loc), Kick_prob_calc/1(R_4_loc)
  Kick_prob_calc/1(kick_direction) -> Display4/1, kick_direction/1
  R_1_sen/1 -> zero_padding/1(u)
  zero_padding/1(y) -> R3_O_dist_val/3(sen_1_val), R4_O_dist_val/3(sen_1_val), R2_O_dist_val/3(sen_1_val)
  R2_O_dist_val/1(y) -> Display/1, Multiply1/1
  R3_O_dist_val/1(y) -> Display1/1, Multiply2/1
  R4_O_dist_val/1(y) -> Display2/1, Multiply/1
  Distance/1(R1_R2_dis) -> Sum/1
  Multiply1/1 -> Sum/2
  Distance1/1(R1_R3_dis) -> Sum1/1
  Distance2/1(R1_R4_dis) -> Sum2/1
  Multiply2/1 -> Sum1/2
  Multiply/1 -> Sum2/2
  Sum/1 -> Kick_prob_calc/4(R1_R2_dis)
  Sum1/1 -> Kick_prob_calc/5(R1_R3_dis)
  Sum2/1 -> Kick_prob_calc/6(R1_R4_dis)

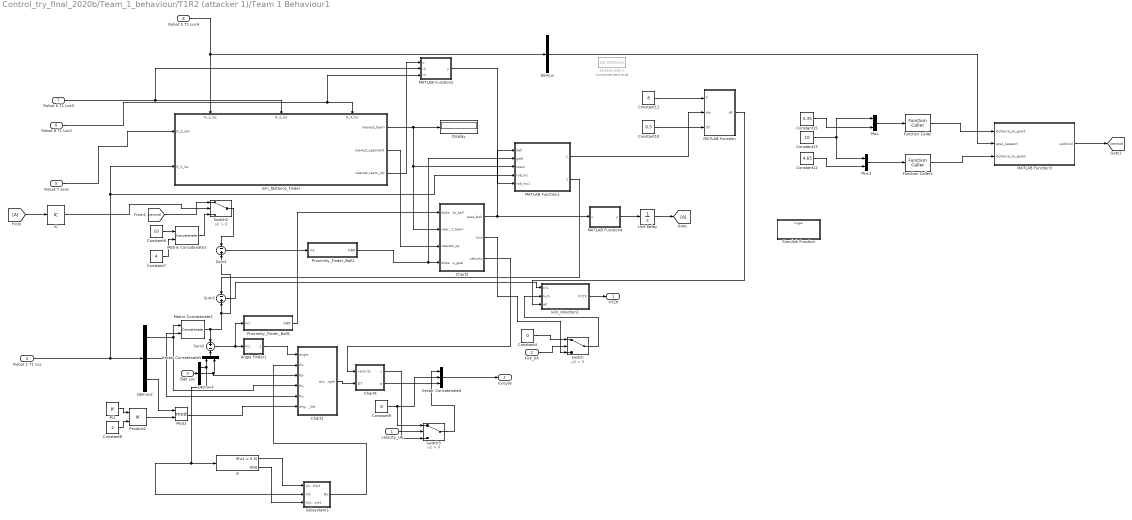
== system Control_try_final_2020b/Team_1_behaviour/T1R2 (attacker 1)/Team 1 Behaviour1 ==
  velocity_UA : Inport
  kick_UA : Inport  Port=2
  Ball Loc : Inport  Port=3
  Robot 1 T1 Loc : Inport  Port=4
  Robot 7 sens : Inport  Port=5
  Robot 8 T1 Loc2 : Inport  Port=6
  Robot 6 T1 Loc3 : Inport  Port=7
  Robot 5 T1 Loc4 : Inport  Port=8
  Angle Finder1 : Subsystem
  Chart1 : Stateflow chart  TreatAsAtomicUnit=on
      settings: PortSchema="{\"entries\":[{\"content\":{\"sides\":[{\"content\":{\"connectorIds\":[\"In5\",\"In1\",\"In2\",\"In3\",\"In4\",\"In6\"]},\"type\":\"ConnectorPlacement.EquallySpacedRectSide\",\"uuid\":\"cd25ea97-6441-4246-83f2-eec847899c89\"},{\"content\":{\"connectorIds\":[\"Out1\"],\"side\":\"RIGHT\"},\"type\":\"ConnectorPlacement.EquallySpacedRectSide\",\"uuid\":\"ef7d77a7-1549-4474-8b84-35bb8af5d0e7\"},{\"content\":{\"connectorIds\":[],\"side\":\"TOP\"},\"type\":\"ConnectorPlacement.EquallySpacedRectSide\",\"uuid\":\"0f0ce596-3061-42ac-890a-62bc4f21ac3e\"},{\"content\":{\"connectorIds\":[],\"side\":\"BOTTOM\"},\"type\":\"ConnectorPlacement.EquallySpacedRectSide\",\"uuid\":\"682b3de5-e999-4954-b7ff-f16ecbf9ea8f\"}]},\"type\":\"ConnectorPlacement.EquallySpacedConnector\",\"uuid\":\"15dca8e2-6a60-4a0d-80a5-3c295a61c828\"}],\"packageUris\":[\"http://schema.mathworks.com/mf0/Connector/R2020b\"],\"version\":\"1.0\"}"
  Chart2 : Stateflow chart  TreatAsAtomicUnit=on
      settings: PortSchema="{\"entries\":[{\"content\":{\"sides\":[{\"content\":{\"connectorIds\":[\"In1\",\"In2\",\"In3\",\"In4\"]},\"type\":\"ConnectorPlacement.EquallySpacedRectSide\",\"uuid\":\"0588d813-8053-43c2-aa9d-d3a846613814\"},{\"content\":{\"connectorIds\":[\"Out3\",\"Out1\",\"Out2\"],\"side\":\"RIGHT\"},\"type\":\"ConnectorPlacement.EquallySpacedRectSide\",\"uuid\":\"b273383a-6a54-4b9f-9eb1-40fc7adfc00e\"},{\"content\":{\"connectorIds\":[],\"side\":\"TOP\"},\"type\":\"ConnectorPlacement.EquallySpacedRectSide\",\"uuid\":\"d9b37716-6c8a-415a-a248-7c4c2a5acdca\"}]},\"type\":\"ConnectorPlacement.EquallySpacedConnector\",\"uuid\":\"4383e6fa-6fc5-4afb-a6cc-0c4f83dd9bd6\"}],\"packageUris\":[\"http://schema.mathworks.com/mf0/Connector/R2020b\"],\"version\":\"1.0\"}"
  Chart4 : Stateflow chart  TreatAsAtomicUnit=on
  Constant10 : Constant  Value=0.5
  Constant11 : Constant  Value=8
  Constant12 : Constant  Value=4.65
  Constant13 : Constant  Value=10
  Constant15 : Constant  Value=3.35
  Constant4 : Constant  Value=0
  Constant6 : Constant  Value=10
  Constant7 : Constant  Value=4
  Constant8 : Constant  Value=2
  Constant9 : Constant  Value=0
  Demux : Demux  Outputs=3
  Demux2 : Demux  Outputs=3
  Demux4 : Demux  Outputs=3
  Display : Display
  Function Caller : FunctionCaller  FunctionPrototype=y = f(u)  InputArgumentSpecifications=<Enter example>  OutputArgumentSpecifications=<Enter example>
  Function Caller1 : FunctionCaller  FunctionPrototype=y = f(u)  InputArgumentSpecifications=<Enter example>  OutputArgumentSpecifications=<Enter example>
  IC : InitialCondition  Value=0
  If : If  IfExpression=u1 < 5.5
  MATLAB Function : MATLAB Function  TreatAsAtomicUnit=on
  MATLAB Function1 : MATLAB Function  TreatAsAtomicUnit=on
  MATLAB Function2 : MATLAB Function  TreatAsAtomicUnit=on
  MATLAB Function3 : MATLAB Function  TreatAsAtomicUnit=on
  MATLAB Function4 : MATLAB Function  TreatAsAtomicUnit=on
  Matrix Concatenate1 : Concatenate  Mode=Multidimensional array  ConcatenateDimension=2
  Matrix Concatenate2 : Concatenate  Mode=Multidimensional array  ConcatenateDimension=2
  Mod1 : Math  Operator=mod  SaturateOnIntegerOverflow=on
  Mux : Mux  Inputs=2
  Mux1 : Mux  Inputs=2
  Pi1 : Constant  Value=pi  OutDataTypeStr=Inherit: Inherit via back propagation
  Product2 : Product
  Proximity_Finder_Ball1 : Subsystem
  Proximity_Finder_Ball2 : Subsystem
  Simulink Function : Subsystem  TreatAsAtomicUnit=on
  Subsystem1 : Subsystem
  Sum2 : Sum  Inputs=+-
  Sum3 : Sum  Inputs=-+
  Sum4 : Sum  Inputs=-+
  Switch : Switch  Criteria=u2 > Threshold
  Switch2 : Switch  Criteria=u2 > Threshold
  Switch3 : Switch  Criteria=u2 > Threshold
  Unit Delay : UnitDelay  SampleTime=-1  HasFrameUpgradeWarning=on
  Vector Concatenate4 : Concatenate  NumInputs=3
  Vector Concatenate5 : Concatenate
  kickForceSim : FromWorkspace  Commented=on  VariableName=out.KickForce
  kick_direction1 : Subsystem
  min_Distance_Finder : Subsystem
      settings: PortSchema="{\"entries\":[{\"content\":{\"sides\":[{\"content\":{\"connectorIds\":[\"In1\",\"In2\"]},\"type\":\"ConnectorPlacement.EquallySpacedRectSide\",\"uuid\":\"45cf91c7-7d38-4a19-bf35-d1d31095287a\"},{\"content\":{\"connectorIds\":[\"Out1\",\"Out2\",\"Out3\"],\"side\":\"RIGHT\"},\"type\":\"ConnectorPlacement.EquallySpacedRectSide\",\"uuid\":\"645394ba-2e5d-4060-b61c-cc9330ee0038\"},{\"content\":{\"connectorIds\":[\"In3\",\"In4\",\"In5\"],\"side\":\"TOP\"},\"type\":\"ConnectorPlacement.EquallySpacedRectSide\",\"uuid\":\"4fc56b73-04ec-476f-b487-f0e593f708ad\"},{\"content\":{\"connectorIds\":[],\"side\":\"BOTTOM\"},\"type\":\"ConnectorPlacement.EquallySpacedRectSide\",\"uuid\":\"cd306436-fd63-4e79-88e6-7a63c0840ed7\"}]},\"type\":\"ConnectorPlacement.EquallySpacedConnector\",\"uuid\":\"5cf2ee04-00eb-490b-958c-5fb90b43d325\"}],\"packageUris\":[\"http://schema.mathworks.com/mf0/Connector/R2020b\"],\"version\":\"1.0\"}"
  XYZK : Outport
  VxVyW : Outport  Port=2
  wires:
  Constant4/1 -> Switch/1
  kick_UA/1 -> Switch/2
  Subsystem1/1(Bx) -> Chart1/1(Bx)
  Demux4/2 -> Chart1/2(By), Vector Concatenate5/2
  Sum4/1 -> Proximity_Finder_Ball2/1(In1)
  Demux4/1 -> Vector Concatenate5/1, If/1, Subsystem1/2(In2)
  If/2 -> Subsystem1/3(Action Port1)
  Constant13/1 -> Mux1/1, Mux/1
  Constant12/1 -> Mux1/2
  Ball Loc/1 -> Demux4/1
  If/1 -> Subsystem1/1(Action Port)
  Switch2/1 -> Sum4/1
  [centroid] -> Switch2/1
  Mux1/1 -> Function Caller1/1
  Mux/1 -> Function Caller/1
  Matrix Concatenate1/1 -> Switch2/3
  [A] -> IC/1
  Angle Finder1/1(angle) -> Chart1/5(angle)
  MATLAB Function4/1(y) -> Unit Delay/1
  Demux/2 -> MATLAB Function3/2(goal_keeperY)
  Constant11/1 -> MATLAB Function/1(F)
  Function Caller/1 -> MATLAB Function3/1(distance_to_goal1)
  min_Distance_Finder/2(nearest_opponent) -> Chart2/3(nearest_op)
  Chart2/1(kick) -> Switch/3
  Mod1/1 -> Chart1/6(angle_bot)
  Demux2/1 -> Matrix Concatenate2/1, Chart1/3(Rx)
  Constant6/1 -> Matrix Concatenate1/1
  Robot 8 T1 Loc2/1 -> MATLAB Function2/3(r4), min_Distance_Finder/5(R_4_loc)
  MATLAB Function/1(dF) -> kick_direction1/3(dF)
  Product2/1 -> Mod1/2
  min_Distance_Finder/3(nearest_team_idx) -> MATLAB Function2/1(u)
  MATLAB Function2/1(y) -> MATLAB Function1/5(rob_loc1)
  Constant15/1 -> Mux/2
  min_Distance_Finder/1(nearest_team) -> Chart2/2(nearest_team), MATLAB Function1/3(team), Display/1
  Chart4/2(w) -> Vector Concatenate4/3
  Chart2/2(velocity) -> Chart4/1(velocity)
  Sum2/1 -> Proximity_Finder_Ball1/1(In1), Angle Finder1/1(In1)
  IC/1 -> Switch2/2
  Constant8/1 -> Product2/2
  Constant9/1 -> Switch3/1, Vector Concatenate4/2
  Vector Concatenate5/1 -> Sum2/2
  MATLAB Function1/2(z) -> Sum3/1
  Chart1/1(actual_angle) -> Chart4/2(DT)
  Pi1/1 -> Product2/1
  Robot 5 T1 Loc4/1 -> min_Distance_Finder/3(R_1_loc), Demux/1
  Proximity_Finder_Ball1/1(DBR) -> Chart2/1(distance_to_ball)
  Function Caller1/1 -> MATLAB Function3/3(distance_to_goal2)
  Chart4/1(v) -> Switch3/3
  MATLAB Function3/1(centroid) -> [centroid]
  Robot 6 T1 Loc3/1 -> MATLAB Function2/2(r3), min_Distance_Finder/4(R_3_loc)
  Demux2/2 -> Matrix Concatenate2/2, Chart1/4(Ry)
  Constant10/1 -> MATLAB Function/3(dT)
  Unit Delay/1 -> [A]
  Demux2/3 -> Mod1/1
  MATLAB Function1/1(y) -> MATLAB Function/2(dis)
  Robot 7 sens/1 -> min_Distance_Finder/1(R_2_sen)
  Matrix Concatenate2/1 -> Sum4/2, Sum3/2, Sum2/1
  Proximity_Finder_Ball2/1(DBR) -> MATLAB Function1/2(goal), Chart2/4(distance_to_goal)
  Chart2/3(pass_beh) -> MATLAB Function1/1(beh), MATLAB Function4/1(u)
  kick_direction1/1(XYZK) -> XYZK/1
  Constant7/1 -> Matrix Concatenate1/2
  Vector Concatenate4/1 -> VxVyW/1
  Sum3/1 -> kick_direction1/1(In1)
  Robot 1 T1 Loc/1 -> MATLAB Function1/4(rob_loc), min_Distance_Finder/2(R_2_loc), Demux2/1
  Switch3/1 -> Vector Concatenate4/1
  velocity_UA/1 -> Switch3/2
  Switch/1 -> kick_direction1/2(kick)

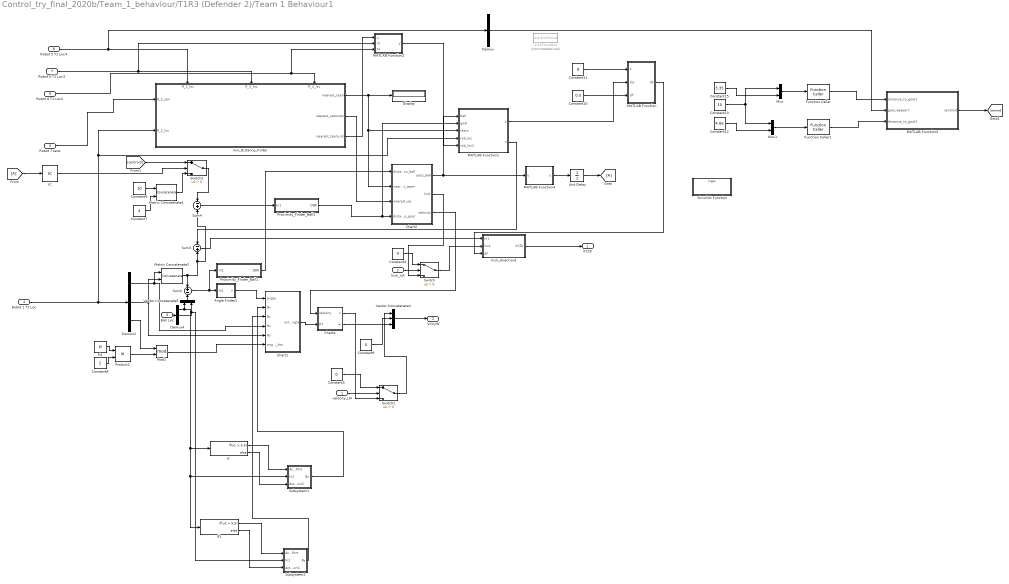
== system Control_try_final_2020b/Team_1_behaviour/T1R3 (Defender 2)/Team 1 Behaviour1 ==
  velocity_UA : Inport
  kick_UA : Inport  Port=2
  Ball Loc : Inport  Port=3
  Robot 1 T1 Loc : Inport  Port=4
  Robot 7 sens : Inport  Port=5
  Robot 8 T1 Loc2 : Inport  Port=6
  Robot 6 T1 Loc3 : Inport  Port=7
  Robot 5 T1 Loc4 : Inport  Port=8
  Angle Finder1 : Subsystem
  Chart1 : Stateflow chart  TreatAsAtomicUnit=on
      settings: PortSchema="{\"entries\":[{\"content\":{\"sides\":[{\"content\":{\"connectorIds\":[\"In5\",\"In1\",\"In2\",\"In3\",\"In4\",\"In6\"]},\"type\":\"ConnectorPlacement.EquallySpacedRectSide\",\"uuid\":\"cd25ea97-6441-4246-83f2-eec847899c89\"},{\"content\":{\"connectorIds\":[\"Out1\"],\"side\":\"RIGHT\"},\"type\":\"ConnectorPlacement.EquallySpacedRectSide\",\"uuid\":\"ef7d77a7-1549-4474-8b84-35bb8af5d0e7\"},{\"content\":{\"connectorIds\":[],\"side\":\"TOP\"},\"type\":\"ConnectorPlacement.EquallySpacedRectSide\",\"uuid\":\"0f0ce596-3061-42ac-890a-62bc4f21ac3e\"},{\"content\":{\"connectorIds\":[],\"side\":\"BOTTOM\"},\"type\":\"ConnectorPlacement.EquallySpacedRectSide\",\"uuid\":\"682b3de5-e999-4954-b7ff-f16ecbf9ea8f\"}]},\"type\":\"ConnectorPlacement.EquallySpacedConnector\",\"uuid\":\"15dca8e2-6a60-4a0d-80a5-3c295a61c828\"}],\"packageUris\":[\"http://schema.mathworks.com/mf0/Connector/R2020b\"],\"version\":\"1.0\"}"
  Chart2 : Stateflow chart  TreatAsAtomicUnit=on
      settings: PortSchema="{\"entries\":[{\"content\":{\"sides\":[{\"content\":{\"connectorIds\":[\"In1\",\"In2\",\"In3\",\"In4\"]},\"type\":\"ConnectorPlacement.EquallySpacedRectSide\",\"uuid\":\"0588d813-8053-43c2-aa9d-d3a846613814\"},{\"content\":{\"connectorIds\":[\"Out3\",\"Out1\",\"Out2\"],\"side\":\"RIGHT\"},\"type\":\"ConnectorPlacement.EquallySpacedRectSide\",\"uuid\":\"b273383a-6a54-4b9f-9eb1-40fc7adfc00e\"},{\"content\":{\"connectorIds\":[],\"side\":\"TOP\"},\"type\":\"ConnectorPlacement.EquallySpacedRectSide\",\"uuid\":\"d9b37716-6c8a-415a-a248-7c4c2a5acdca\"}]},\"type\":\"ConnectorPlacement.EquallySpacedConnector\",\"uuid\":\"4383e6fa-6fc5-4afb-a6cc-0c4f83dd9bd6\"}],\"packageUris\":[\"http://schema.mathworks.com/mf0/Connector/R2020b\"],\"version\":\"1.0\"}"
  Chart4 : Stateflow chart  TreatAsAtomicUnit=on
  Constant10 : Constant  Value=0.5
  Constant11 : Constant  Value=8
  Constant12 : Constant  Value=4.65
  Constant13 : Constant  Value=10
  Constant15 : Constant  Value=3.35
  Constant4 : Constant  Value=0
  Constant5 : Constant  Value=0
  Constant6 : Constant  Value=10
  Constant7 : Constant  Value=4
  Constant8 : Constant  Value=2
  Constant9 : Constant  Value=0
  Demux : Demux  Outputs=3
  Demux2 : Demux  Outputs=3
  Demux4 : Demux  Outputs=3
  Display : Display
  Function Caller : FunctionCaller  FunctionPrototype=y = f(u)  InputArgumentSpecifications=<Enter example>  OutputArgumentSpecifications=<Enter example>
  Function Caller1 : FunctionCaller  FunctionPrototype=y = f(u)  InputArgumentSpecifications=<Enter example>  OutputArgumentSpecifications=<Enter example>
  IC : InitialCondition  Value=0
  If : If  IfExpression=u1 > 5.5
  If1 : If  IfExpression=u1 > 5.5
  MATLAB Function : MATLAB Function  TreatAsAtomicUnit=on
  MATLAB Function1 : MATLAB Function  TreatAsAtomicUnit=on
  MATLAB Function2 : MATLAB Function  TreatAsAtomicUnit=on
  MATLAB Function3 : MATLAB Function  TreatAsAtomicUnit=on
  MATLAB Function4 : MATLAB Function  TreatAsAtomicUnit=on
  Matrix Concatenate1 : Concatenate  Mode=Multidimensional array  ConcatenateDimension=2
  Matrix Concatenate2 : Concatenate  Mode=Multidimensional array  ConcatenateDimension=2
  Mod1 : Math  Operator=mod  SaturateOnIntegerOverflow=on
  Mux : Mux  Inputs=2
  Mux1 : Mux  Inputs=2
  Pi1 : Constant  Value=pi  OutDataTypeStr=Inherit: Inherit via back propagation
  Product2 : Product
  Proximity_Finder_Ball1 : Subsystem
  Proximity_Finder_Ball2 : Subsystem
  Simulink Function : Subsystem  TreatAsAtomicUnit=on
  Subsystem1 : Subsystem
  Subsystem2 : Subsystem
  Sum2 : Sum  Inputs=+-
  Sum3 : Sum  Inputs=-+
  Sum4 : Sum  Inputs=-+
  Switch : Switch  Criteria=u2 > Threshold
  Switch1 : Switch  Criteria=u2 > Threshold
  Switch2 : Switch  Criteria=u2 > Threshold
  Unit Delay : UnitDelay  SampleTime=-1  HasFrameUpgradeWarning=on
  Vector Concatenate4 : Concatenate  NumInputs=3
  Vector Concatenate5 : Concatenate
  kickForceSim : FromWorkspace  Commented=on  VariableName=out.KickForce
  kick_direction1 : Subsystem
  min_Distance_Finder : Subsystem
      settings: PortSchema="{\"entries\":[{\"content\":{\"sides\":[{\"content\":{\"connectorIds\":[\"In1\",\"In2\"]},\"type\":\"ConnectorPlacement.EquallySpacedRectSide\",\"uuid\":\"45cf91c7-7d38-4a19-bf35-d1d31095287a\"},{\"content\":{\"connectorIds\":[\"Out1\",\"Out2\",\"Out3\"],\"side\":\"RIGHT\"},\"type\":\"ConnectorPlacement.EquallySpacedRectSide\",\"uuid\":\"645394ba-2e5d-4060-b61c-cc9330ee0038\"},{\"content\":{\"connectorIds\":[\"In3\",\"In4\",\"In5\"],\"side\":\"TOP\"},\"type\":\"ConnectorPlacement.EquallySpacedRectSide\",\"uuid\":\"4fc56b73-04ec-476f-b487-f0e593f708ad\"},{\"content\":{\"connectorIds\":[],\"side\":\"BOTTOM\"},\"type\":\"ConnectorPlacement.EquallySpacedRectSide\",\"uuid\":\"cd306436-fd63-4e79-88e6-7a63c0840ed7\"}]},\"type\":\"ConnectorPlacement.EquallySpacedConnector\",\"uuid\":\"5cf2ee04-00eb-490b-958c-5fb90b43d325\"}],\"packageUris\":[\"http://schema.mathworks.com/mf0/Connector/R2020b\"],\"version\":\"1.0\"}"
  XYZK : Outport
  VxVyW : Outport  Port=2
  wires:
  kick_direction1/1(XYZK) -> XYZK/1
  Constant4/1 -> Switch/1
  kick_UA/1 -> Switch/2
  Constant5/1 -> Switch1/1
  velocity_UA/1 -> Switch1/2
  MATLAB Function4/1(y) -> Unit Delay/1
  If1/2 -> Subsystem2/3(Action Port1)
  Constant6/1 -> Matrix Concatenate1/1
  Constant9/1 -> Vector Concatenate4/2
  Demux4/1 -> If1/1, Subsystem1/2(In2), If/1, Vector Concatenate5/1
  Matrix Concatenate2/1 -> Sum4/2, Sum3/2, Sum2/1
  Chart1/1(actual_angle) -> Chart4/2(DT)
  Subsystem1/1(Bx) -> Chart1/1(Bx)
  Demux2/3 -> Mod1/1
  Constant8/1 -> Product2/2
  If/2 -> Subsystem1/3(Action Port1)
  Sum3/1 -> kick_direction1/1(In1)
  Robot 6 T1 Loc3/1 -> MATLAB Function2/2(r3), min_Distance_Finder/4(R_3_loc)
  Demux4/2 -> Subsystem2/2(In2), Vector Concatenate5/2
  Proximity_Finder_Ball2/1(DBR) -> MATLAB Function1/2(goal), Chart2/4(distance_to_goal)
  min_Distance_Finder/3(nearest_team_idx) -> MATLAB Function2/1(u)
  If1/1 -> Subsystem2/1(Action Port)
  If/1 -> Subsystem1/1(Action Port)
  Pi1/1 -> Product2/1
  Function Caller1/1 -> MATLAB Function3/3(distance_to_goal2)
  Chart4/2(w) -> Vector Concatenate4/3
  Ball Loc/1 -> Demux4/1
  Robot 8 T1 Loc2/1 -> MATLAB Function2/3(r4), min_Distance_Finder/5(R_4_loc)
  [A] -> IC/1
  Robot 7 sens/1 -> min_Distance_Finder/1(R_2_sen)
  Constant15/1 -> Mux/2
  Mod1/1 -> Chart1/6(angle_bot)
  Sum2/1 -> Proximity_Finder_Ball1/1(In1), Angle Finder1/1(In1)
  Robot 1 T1 Loc/1 -> MATLAB Function1/4(rob_loc), min_Distance_Finder/2(R_2_loc), Demux2/1
  Demux/2 -> MATLAB Function3/2(goal_keeperY)
  Constant13/1 -> Mux1/1, Mux/1
  MATLAB Function1/1(y) -> MATLAB Function/2(dis)
  Demux2/2 -> Matrix Concatenate2/2, Chart1/4(Ry)
  MATLAB Function1/2(z) -> Sum3/1
  Unit Delay/1 -> [A]
  Chart2/3(pass_beh) -> MATLAB Function1/1(beh), MATLAB Function4/1(u)
  Vector Concatenate4/1 -> VxVyW/1
  Constant12/1 -> Mux1/2
  Proximity_Finder_Ball1/1(DBR) -> Chart2/1(distance_to_ball)
  Mux1/1 -> Function Caller1/1
  Mux/1 -> Function Caller/1
  Constant10/1 -> MATLAB Function/3(dT)
  Sum4/1 -> Proximity_Finder_Ball2/1(In1)
  MATLAB Function3/1(centroid) -> [centroid]
  Switch2/1 -> Sum4/1
  min_Distance_Finder/1(nearest_team) -> Chart2/2(nearest_team), MATLAB Function1/3(team), Display/1
  min_Distance_Finder/2(nearest_opponent) -> Chart2/3(nearest_op)
  Chart4/1(v) -> Switch1/3
  Chart2/2(velocity) -> Chart4/1(velocity)
  Subsystem2/1(By) -> Chart1/2(By)
  Chart2/1(kick) -> Switch/3
  Function Caller/1 -> MATLAB Function3/1(distance_to_goal1)
  Angle Finder1/1(angle) -> Chart1/5(angle)
  Product2/1 -> Mod1/2
  MATLAB Function/1(dF) -> kick_direction1/3(dF)
  Matrix Concatenate1/1 -> Switch2/3
  Robot 5 T1 Loc4/1 -> Demux/1, min_Distance_Finder/3(R_1_loc)
  MATLAB Function2/1(y) -> MATLAB Function1/5(rob_loc1)
  Constant11/1 -> MATLAB Function/1(F)
  Demux2/1 -> Matrix Concatenate2/1, Chart1/3(Rx)
  Constant7/1 -> Matrix Concatenate1/2
  IC/1 -> Switch2/2
  Vector Concatenate5/1 -> Sum2/2
  [centroid] -> Switch2/1
  Switch/1 -> kick_direction1/2(kick)
  Switch1/1 -> Vector Concatenate4/1
